simulink model "statcom"  (R2022a)
settings: Solver=VariableStepAuto  StartTime=0.0  StopTime=10.0  RelTol=1e-3
libraries: spsSeriesRLCBranchLib x10, spsIGBTDiodeLib x6, spsThreePhaseVIMeasurementLib x3, spsThreePhaseParallelRLCLoadLib x1, spsThreePhaseSourceLib x1, spsVoltageMeasurementLib x1
settings Model: Creator=neshan  LastModifiedBy=neshan

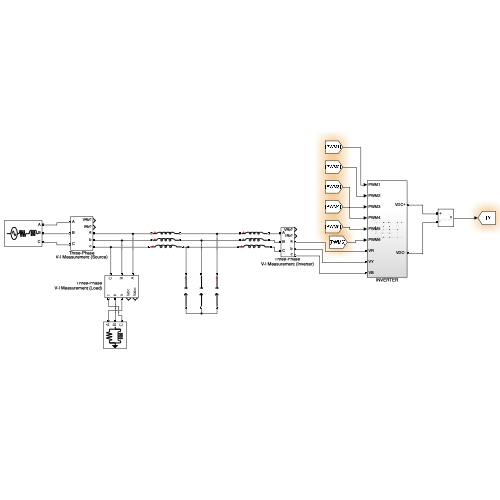
[thumbnail: Simulink's stored preview of the top-level diagram]
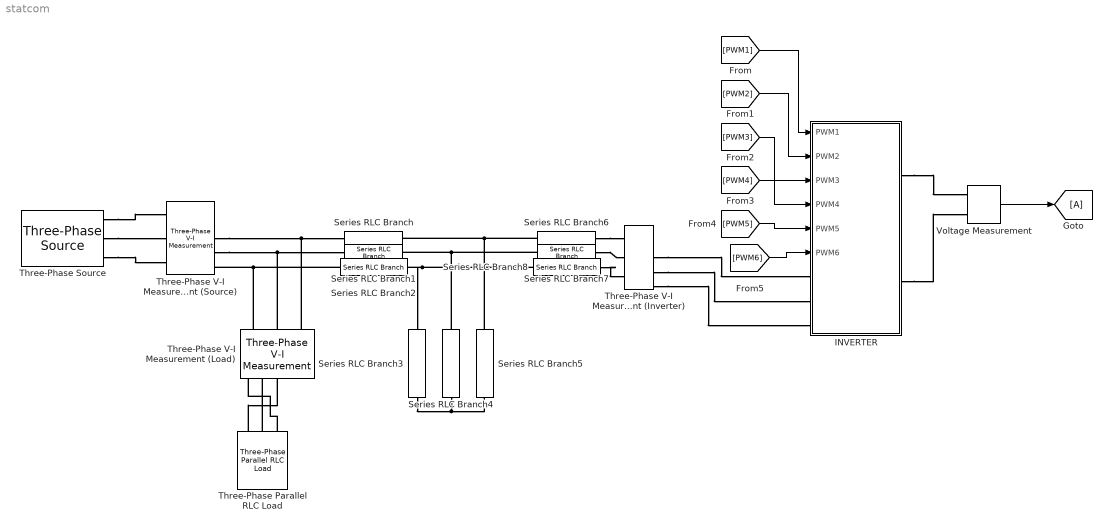
== system statcom ==
  Goto : Goto
  INVERTER : Subsystem
  Series RLC Branch{,1..2,6..8} (6 alike) : spsSeriesRLCBranchLib/Series RLC Branch  LConnTagsString=__new0  RConnTagsString=__new0  BranchType=L  Resistance=1  Inductance=500e-6  SetiL0=off  InitialCurrent=0  Capacitance=1e-6  Setx0=off  InitialVoltage=0  Measurements=None
  Series RLC Branch3 : spsSeriesRLCBranchLib/Series RLC Branch  LConnTagsString=__new0  RConnTagsString=__new0  BranchType=C  Resistance=1  Inductance=500e-6  SetiL0=off  InitialCurrent=0  Capacitance=100e-6  Setx0=off  InitialVoltage=0  Measurements=None
  Series RLC Branch4 : spsSeriesRLCBranchLib/Series RLC Branch  LConnTagsString=__new0  RConnTagsString=__new0  BranchType=C  Resistance=1  Inductance=500e-6  SetiL0=off  InitialCurrent=0  Capacitance=100e-6  Setx0=off  InitialVoltage=0  Measurements=None
  Series RLC Branch5 : spsSeriesRLCBranchLib/Series RLC Branch  LConnTagsString=__new0  RConnTagsString=__new0  BranchType=C  Resistance=1  Inductance=500e-6  SetiL0=off  InitialCurrent=0  Capacitance=100e-6  Setx0=off  InitialVoltage=0  Measurements=None
  Three-Phase Parallel RLC Load : spsThreePhaseParallelRLCLoadLib/Three-Phase Parallel RLC Load  LConnTagsString=A|B|C  Configuration=Y (grounded)  NominalVoltage=415  Vabc=[1e3 1e3 1e3]  Vabcp=[1e3 1e3 1e3]  NominalFrequency=50  UnbalancedPower=off  ActivePower=200e3  InductivePower=100e3  CapacitivePower=0  Pabc=[10e3 9e3 11e3]  QLabc=[100 90 110]  QCabc=[100 90 110]  Pabcp=[10e3 9e3 11e3]  QLabcp=[100 90 110]  QCabcp=[100 90 110]  Measurements=None  LoadType=constant Z
  Three-Phase V-I Measurement (Inverter) : spsThreePhaseVIMeasurementLib/Three-Phase V-I Measurement  VoltageMeasurement=phase-to-ground  SetLabelV=off  LabelV=Vabc  Vpu=off  VpuLL=off  CurrentMeasurement=yes  SetLabelI=off  LabelI=Iabc  Ipu=off  Pbase=100e6  Vbase=500e3  OutputType=Complex  PhasorSimulation=off  PSBequivalent=0
  Three-Phase V-I Measurement (Load) : spsThreePhaseVIMeasurementLib/Three-Phase V-I Measurement  VoltageMeasurement=phase-to-ground  SetLabelV=off  LabelV=Vabc  Vpu=off  VpuLL=off  CurrentMeasurement=yes  SetLabelI=off  LabelI=Iabc  Ipu=off  Pbase=100e6  Vbase=500e3  OutputType=Complex  PhasorSimulation=off  PSBequivalent=0
  Three-Phase V-I Measurement (Source) : spsThreePhaseVIMeasurementLib/Three-Phase V-I Measurement  VoltageMeasurement=phase-to-ground  SetLabelV=off  LabelV=Vabc  Vpu=off  VpuLL=off  CurrentMeasurement=yes  SetLabelI=off  LabelI=Iabc  Ipu=off  Pbase=100e6  Vbase=500e3  OutputType=Complex  PhasorSimulation=off  PSBequivalent=0
  Three-Phase Source : spsThreePhaseSourceLib/Three-Phase Source  InternalConnection=Y  VoltagePhases=off  Voltage=415  PhaseAngle=0  Voltage_phases=[25e3 25e3 25e3]/sqrt(3)  PhaseAngles_phases=[0 -120 +120]  Frequency=50  NonIdealSource=on  SpecifyImpedance=off  Resistance=1e-6  Inductance=1e-6  ShortCircuitLevel=100e6  BaseVoltage=415  XRratio=7  BusType=swing  Pref=10e3  Qref=0  Prefabc=[10e3, 10e3, 10e3]  Qrefabc=[0, 0, 0]  Qmin=-inf  Qmax=inf
  Voltage Measurement : spsVoltageMeasurementLib/Voltage Measurement  PhasorSimulation=off  OutputType=Complex  PSBequivalent=0
  wires:
  [PWM1] -> INVERTER/1(PWM1)
  [PWM2] -> INVERTER/2(PWM2)
  [PWM3] -> INVERTER/3(PWM3)
  [PWM4] -> INVERTER/4(PWM4)
  [PWM5] -> INVERTER/5(PWM5)
  [PWM6] -> INVERTER/6(PWM6)
  Voltage Measurement/1 -> Goto/1
  connections:
  Three-Phase Source/RConn1 -- Three-Phase V-I Measurement (Source)/LConn1
  Three-Phase Source/RConn2 -- Three-Phase V-I Measurement (Source)/LConn2
  Three-Phase Source/RConn3 -- Three-Phase V-I Measurement (Source)/LConn3
  Series RLC Branch2/LConn1 -- Three-Phase V-I Measurement (Source)/RConn3 -- Three-Phase V-I Measurement (Load)/LConn3
  Three-Phase V-I Measurement (Source)/RConn2 -- Three-Phase V-I Measurement (Load)/LConn2 -- Series RLC Branch1/LConn1
  Three-Phase V-I Measurement (Source)/RConn1 -- Three-Phase V-I Measurement (Load)/LConn1 -- Series RLC Branch/LConn1
  Three-Phase Parallel RLC Load/LConn1 -- Three-Phase V-I Measurement (Load)/RConn1
  Three-Phase Parallel RLC Load/LConn2 -- Three-Phase V-I Measurement (Load)/RConn2
  Three-Phase Parallel RLC Load/LConn3 -- Three-Phase V-I Measurement (Load)/RConn3
  Series RLC Branch2/RConn1 -- Series RLC Branch3/LConn1 -- Series RLC Branch8/LConn1
  Series RLC Branch4/LConn1 -- Series RLC Branch7/LConn1 -- Series RLC Branch1/RConn1
  Series RLC Branch5/LConn1 -- Series RLC Branch/RConn1 -- Series RLC Branch6/LConn1
  Series RLC Branch3/RConn1 -- Series RLC Branch4/RConn1 -- Series RLC Branch5/RConn1
  Series RLC Branch6/RConn1 -- Three-Phase V-I Measurement (Inverter)/LConn1
  Series RLC Branch7/RConn1 -- Three-Phase V-I Measurement (Inverter)/LConn2
  Series RLC Branch8/RConn1 -- Three-Phase V-I Measurement (Inverter)/LConn3
  Three-Phase V-I Measurement (Inverter)/RConn1 -- INVERTER/LConn1
  Three-Phase V-I Measurement (Inverter)/RConn2 -- INVERTER/LConn2
  Three-Phase V-I Measurement (Inverter)/RConn3 -- INVERTER/LConn3
  INVERTER/RConn1 -- Voltage Measurement/LConn1
  INVERTER/RConn2 -- Voltage Measurement/LConn2

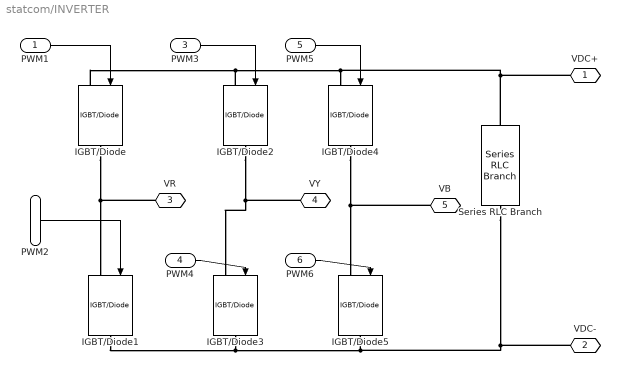
== system statcom/INVERTER ==
  PWM1 : Inport
  PWM2 : Inport  Port=2
  PWM3 : Inport  Port=3
  PWM4 : Inport  Port=4
  PWM5 : Inport  Port=5
  PWM6 : Inport  Port=6
  IGBT/Diode{,1..5} (6 alike) : spsIGBTDiodeLib/IGBT//Diode  Ron=1e-3  Rs=1e5  Cs=inf  Measurements=off
  Series RLC Branch : spsSeriesRLCBranchLib/Series RLC Branch  LConnTagsString=__new0  RConnTagsString=__new0  BranchType=RC  Resistance=1e-3  Inductance=1e-3  SetiL0=off  InitialCurrent=0  Capacitance=5600e-6  Setx0=off  InitialVoltage=0  Measurements=None
  VDC+ : PMIOPort  Side=Right
  VDC- : PMIOPort  Port=2  Side=Right
  VR : PMIOPort  Port=3  Side=Left
  VY : PMIOPort  Port=4  Side=Left
  VB : PMIOPort  Port=5  Side=Left
  wires:
  PWM2/1 -> IGBT/Diode1/1
  PWM5/1 -> IGBT/Diode4/1
  PWM6/1 -> IGBT/Diode5/1
  PWM3/1 -> IGBT/Diode2/1
  PWM4/1 -> IGBT/Diode3/1
  PWM1/1 -> IGBT/Diode/1
  connections:
  IGBT/Diode4/RConn1 -- VB/RConn1 -- IGBT/Diode5/LConn1
  IGBT/Diode1/RConn1 -- IGBT/Diode3/RConn1 -- VDC-/RConn1 -- Series RLC Branch/RConn1 -- IGBT/Diode5/RConn1
  IGBT/Diode2/RConn1 -- VY/RConn1 -- IGBT/Diode3/LConn1
  IGBT/Diode/RConn1 -- VR/RConn1 -- IGBT/Diode1/LConn1
  IGBT/Diode/LConn1 -- IGBT/Diode2/LConn1 -- VDC+/RConn1 -- Series RLC Branch/LConn1 -- IGBT/Diode4/LConn1
